simulink model "Tiefpassfilter"  (Simulink 7.4)
settings: Solver=ode45  StartTime=0.0  StopTime=10.0  RelTol=1e-3
undefined symbols (not defined in the file or in its folder): DiscIntNeverNeededParam, K
settings Model: Creator=roczit00  LastModifiedBy=roczit00

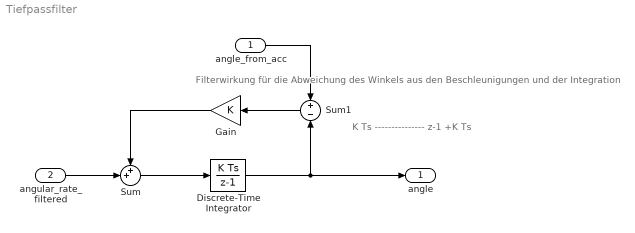
== system Tiefpassfilter ==
  note: K Ts
      | ---------------
      | z-1 +K Ts
  note: Filterwirkung für die
      | Abweichung des Winkels
      | aus den Beschleunigungen
      | und der Integration
  angle_from_acc : Inport  OutDataType=fixdt(1, 16)  OutScaling=2^0
  angular_rate_filtered : Inport  Port=2  OutDataType=fixdt(1, 16)  OutScaling=2^0
  Discrete-Time Integrator : DiscreteIntegrator  OutDataType=fixdt(1, 16)  OutScaling=2^0  ICPrevOutput=DiscIntNeverNeededParam  ICPrevScaledInput=DiscIntNeverNeededParam
  Gain : Gain  Gain=K  ParameterDataType=fixdt(1, 16)  ParameterScaling=2^0  OutDataType=fixdt(1, 16)  OutScaling=2^0
  Sum : Sum  Inputs=++|  OutDataType=fixdt(1, 16)  OutScaling=2^0
  Sum1 : Sum  Inputs=+|-  OutDataType=fixdt(1, 16)  OutScaling=2^0
  angle : Outport  OutDataType=fixdt(1, 16)  OutScaling=2^0
  wires:
  Gain/1 -> Sum/1
  Sum/1 -> Discrete-Time Integrator/1
  angle_from_acc/1 -> Sum1/1
  Sum1/1 -> Gain/1
  Discrete-Time Integrator/1 -> Sum1/2, angle/1
  angular_rate_filtered/1 -> Sum/2
